simulink model "irep_force_control_simu"  (Simulink 8.5)
settings: Solver=ode3  StartTime=0.0  StopTime=inf  FixedStep=dt  RelTol=1e-3
InitFcn:
  | IREP_DEPENDENCY
  | init_omni
  | init_filters
  | init_invivo
  | init_telemanipulation
  | init_parker_xyz
  | init_magnetic_tracker
  | init_loadcell
  | init_scopes
  | init_homing
  | init_force_control
  | init_xpc_invivo_simu
undefined symbols (not defined in the file): ang_vel_scale, B_simu, beta, camera_home_voltage, counter_offset, dt, dt_trakstar, E_Y, encoder_counts, epsilon_robust_inverse, gear_ratio, HomingFineEps, HomingRoughEps, HomingRoughVelocity, I1_primary, I1_secondary, I2_primary, I2_secondary, irep_parameters_left, irep_parameters_right, joystick_filter_coeffs, K_d, K_i, K_naive_inv, K_p, k_right, L1l, L1r, L2l, L2r, L_zeus, left_arm_home_voltage, left_x0_parallelogram, LeftArmHomingDirectionVector, LeftArmHomingIntGain, lin_vel_scale, LOADCELL_BIAS, LOADCELL_GAIN, max_conf_space_speed, N_joystick, N_pots, N_trakstar, OmegaMax, OmegaMin, orientation_epsilon, position_epsilon, pots_filter_coeffs, q_eps_backlash, quadrature_mode, r, right_arm_home_voltage, RightArmHomingDirectionVector, RightArmHomingIntGain, screw_pitch, statics_param, tau_compression_bias, tau_compression_gains, tau_neutral_deadband, tau_tension_bias, tau_tension_gains ... (+14)
libraries: slrtlib x38, xpcrtudplib x13, xpcobsoletelib x13, simulink x6, dspswit3 x2, dspsigops x1
(part 2 of 6)

== system irep_force_control_simu/Joint Level PID Control in mm/PID Compensator ==
  e : Inport
  Enable : EnablePort  StatesWhenEnabling=reset
  Add : Sum  Inputs=+++
  Discrete Derivative : simulink/Discrete/Discrete Derivative  gainval=1.0  ICPrevScaledInput=0.0  InputProcessing=Inherited  OutMin=[]  OutMax=[]  OutDataType=sfix(16)  OutScaling=2^-10  DoSatur=off
  Discrete-Time Integrator : DiscreteIntegrator  SampleTime=dt
  Integral Sat : Saturate  UpperLimit=5  LowerLimit=-5
  Kd : Gain  Gain=K_d  SampleTime=dt
  Ki : Gain  Gain=K_i  SampleTime=dt
  Kp : Gain  Gain=K_p  SampleTime=dt
  Saturation : Saturate  UpperLimit=10  LowerLimit=-10
  u : Outport  InitialOutput=zeros(23,1)
  wires:
  Discrete Derivative/1 -> Add/3
  Kd/1 -> Discrete Derivative/1
  Integral Sat/1 -> Add/2
  Discrete-Time Integrator/1 -> Integral Sat/1
  Saturation/1 -> u/1
  Add/1 -> Saturation/1
  Ki/1 -> Discrete-Time Integrator/1
  Kp/1 -> Add/1
  e/1 -> Ki/1, Kp/1, Kd/1

== system irep_force_control_simu/Scopes/Friction Estimation Data UDP ==
  note: ConfigSpace:
      | b0 [1x1]
      | b1 [2x1]
      | psi [4x1]
      | gamma [1x1]
  note: [9x1]
  note: [4x1]
  note: [6x1]
  note: [6x1]
  note: [6x1]
  note: [6x1]
  sensors : Inport
  ConfigComd : Inport  Port=2
  Clock : Inport  Port=3
  Enable : EnablePort
  Bus Selector1 : BusSelector  OutputSignals=Magnetic Sensors.s1,Magnetic Sensors.s2,Magnetic Sensors.s3,Magnetic Sensors.s4
  Bus Selector2 : BusSelector  OutputSignals=force_sensing.loadcell
  Bus Selector4 : BusSelector  OutputSignals=A/D signals.right arm pots
  Demux : Demux  Outputs=[1 6 1]
  Demux1 : Demux  Outputs=54
  Demux2 : Demux  Outputs=[9 1]
  Mux : Mux  Inputs=10
  Pack : xpcobsoletelib/Utilities/Pack   datatypes={'double' 'double' 'double' 'double' 'double' 'double' 'double' 'double' 'double' 'double' 'double' 'double' 'double' 'double' 'double' 'double' 'double' 'double' 'double' 'double' 'double' 'double' 'double' 'double' 'double' 'double' 'double' 'double' 'double' 'double' 'double' 'double' 'double' 'double' 'double' 'double' 'double' 'double' 'double' 'double' 'double' 'double' 'double' 'double' 'double' 'double' 'double' 'double' 'double' 'double' 'double' 'double' 'double' 'double'}  byteAlign=1
  Rate Transition : RateTransition  OutPortSampleTime=0.012
  Right arm joint def : Subsystem
  STOP : Constant  Value=0
  Send port: 10001 : xpcrtudplib/Legacy UDP/Send   ipAddress=192.168.1.31  ipPort=10001  localPort=-1  vblLen=off  sampletime=0.01
  Terminator : Terminator
  Terminator1 : Terminator
  Terminator2 : Terminator
  wires:
  Pack/1 -> Send port: 10001/1
  sensors/1 -> Right arm joint def/1(sensors), Bus Selector4/1, Bus Selector2/1, Bus Selector1/1
  Bus Selector2/1 -> Mux/3  "<loadcell>"
  Bus Selector1/1 -> Mux/4  "<s1>"
  Bus Selector1/2 -> Mux/5  "<s2>"
  Bus Selector1/3 -> Mux/6  "<s3>"
  Bus Selector1/4 -> Mux/7  "<s4>"
  Right arm joint def/1(right q_cur) -> Mux/1  "q_cur [9x1]"
  ConfigComd/1 -> Demux/1
  Demux/1 -> Terminator/1
  Demux/2 -> Mux/8  "b,psi [6x1]"
  Clock/1 -> Mux/9  "clock [1x1]"
  Mux/1 -> Rate Transition/1
  Demux1/1 -> Pack/1
  Demux1/2 -> Pack/2
  Demux1/3 -> Pack/3
  Demux1/4 -> Pack/4
  Demux1/5 -> Pack/5
  Demux1/6 -> Pack/6
  Demux1/7 -> Pack/7
  Demux1/8 -> Pack/8
  Demux1/9 -> Pack/9
  Demux1/10 -> Pack/10
  Demux1/11 -> Pack/11
  Demux1/12 -> Pack/12
  Demux1/13 -> Pack/13
  Demux1/14 -> Pack/14
  Demux1/15 -> Pack/15
  Demux1/16 -> Pack/16
  Demux1/17 -> Pack/17
  Demux1/18 -> Pack/18
  Demux1/19 -> Pack/19
  Demux1/20 -> Pack/20
  Demux1/21 -> Pack/21
  Demux1/22 -> Pack/22
  Demux1/23 -> Pack/23
  Demux1/24 -> Pack/24
  Demux1/25 -> Pack/25
  Demux1/26 -> Pack/26
  Demux1/27 -> Pack/27
  Demux1/28 -> Pack/28
  Demux1/29 -> Pack/29
  Demux1/30 -> Pack/30
  Demux1/31 -> Pack/31
  Demux1/32 -> Pack/32
  Demux1/33 -> Pack/33
  Demux1/34 -> Pack/34
  Demux1/35 -> Pack/35
  Demux1/36 -> Pack/36
  Demux1/37 -> Pack/37
  Demux1/38 -> Pack/38
  Demux1/39 -> Pack/39
  Demux1/40 -> Pack/40
  Demux1/41 -> Pack/41
  Demux1/42 -> Pack/42
  Demux1/43 -> Pack/43
  Demux1/44 -> Pack/44
  Demux1/45 -> Pack/45
  Demux1/46 -> Pack/46
  Demux1/47 -> Pack/47
  Demux1/48 -> Pack/48
  Demux1/49 -> Pack/49
  Demux1/50 -> Pack/50
  Demux1/51 -> Pack/51
  Demux1/52 -> Pack/52
  Demux1/53 -> Pack/53
  Demux1/54 -> Pack/54
  Rate Transition/1 -> Demux1/1
  STOP/1 -> Mux/10
  Demux/3 -> Terminator1/1
  Bus Selector4/1 -> Demux2/1  "<right arm pots>"
  Demux2/1 -> Mux/2
  Demux2/2 -> Terminator2/1

== system irep_force_control_simu/Scopes/Left arm joint def ==
  In1 : Inport
  Bus Selector5 : BusSelector  OutputSignals=q.Left arm - overall translational movement,q.Left arm - parallelogram insert joint,q.Left arm - parallelogram deployment joint,q.Left arm - proximal segment - bending in X,q.Left arm - proximal segment - bending in Y,q.Left arm - distal segment - bending in x,q.Left arm - distal segment - bending in y,q.Left arm - wrist,q.Left arm - gripper joint
  Mux5 : Mux  Inputs=9
  Out1 : Outport
  wires:
  Bus Selector5/1 -> Mux5/1  "<Left arm - overall translational movement>"
  Bus Selector5/2 -> Mux5/2  "<Left arm - parallelogram insert joint>"
  Bus Selector5/3 -> Mux5/3  "<Left arm - parallelogram deployment joint>"
  Bus Selector5/4 -> Mux5/4  "<Left arm - proximal segment - bending in X>"
  Bus Selector5/5 -> Mux5/5  "<Left arm - proximal segment - bending in Y>"
  Bus Selector5/6 -> Mux5/6  "<Left arm - distal segment - bending in x>"
  Bus Selector5/7 -> Mux5/7  "<Left arm - distal segment - bending in y>"
  Bus Selector5/8 -> Mux5/8  "<Left arm - wrist>"
  Bus Selector5/9 -> Mux5/9  "<Left arm - gripper joint>"
  In1/1 -> Bus Selector5/1
  Mux5/1 -> Out1/1

== system irep_force_control_simu/Scopes/Magnetic Sensor Scopes ==
  In1 : Inport
  Bus Selector4 : BusSelector  OutputSignals=Magnetic Sensors.s1
  Bus Selector5 : BusSelector  OutputSignals=Magnetic Sensors.s2
  Bus Selector6 : BusSelector  OutputSignals=Magnetic Sensors.s3
  Bus Selector7 : BusSelector  OutputSignals=Magnetic Sensors.s4
  Scope M sensor 1 : slrtlib/Displays and Logging/Scope   scopeno=22  scopetype=Host  autostart=on  viewmode=Numerical  formatstr=scope_format_Msensor_1  grid=on  ylimits=[0,0]  nosamples=50  noprepostsamples=0  interleave=1  triggermode=FreeRun  triggersignal=1  trigsignalfromport=off  triggerlevel=0.0  triggerslope=Either  triggerscope=1  triggersample=0  filename=data.dat  mode=Lazy  writesize=512  autorestart=off  dynamicfilemode=off  maxwritefilesize=512*1024^2
  Scope M sensor 2 : slrtlib/Displays and Logging/Scope   scopeno=23  scopetype=Host  autostart=off  viewmode=Numerical  formatstr=scope_format_Msensor_2  grid=on  ylimits=[0,0]  nosamples=50  noprepostsamples=0  interleave=1  triggermode=FreeRun  triggersignal=1  trigsignalfromport=off  triggerlevel=0.0  triggerslope=Either  triggerscope=1  triggersample=0  filename=data.dat  mode=Lazy  writesize=512  autorestart=off  dynamicfilemode=off  maxwritefilesize=512*1024^2
  "Scope M sensor 3 " : slrtlib/Displays and Logging/Scope   scopeno=30  scopetype=Host  autostart=on  viewmode=Numerical  formatstr=scope_format_Msensor_3  grid=on  ylimits=[0,0]  nosamples=50  noprepostsamples=0  interleave=1  triggermode=FreeRun  triggersignal=1  trigsignalfromport=off  triggerlevel=0.0  triggerslope=Either  triggerscope=1  triggersample=0  filename=data.dat  mode=Lazy  writesize=512  autorestart=off  dynamicfilemode=off  maxwritefilesize=512*1024^2
  Scope M sensor 4 : slrtlib/Displays and Logging/Scope   scopeno=31  scopetype=Host  autostart=on  viewmode=Numerical  formatstr=scope_format_Msensor_4  grid=on  ylimits=[0,0]  nosamples=50  noprepostsamples=0  interleave=1  triggermode=FreeRun  triggersignal=1  trigsignalfromport=off  triggerlevel=0.0  triggerslope=Either  triggerscope=1  triggersample=0  filename=data.dat  mode=Lazy  writesize=512  autorestart=off  dynamicfilemode=off  maxwritefilesize=512*1024^2
  wires:
  Bus Selector4/1 -> Scope M sensor 1/1  "<s1>"
  Bus Selector5/1 -> Scope M sensor 2/1  "<s2>"
  Bus Selector6/1 -> "Scope M sensor 3 "/1  "<s3>"
  Bus Selector7/1 -> Scope M sensor 4/1  "<s4>"
  In1/1 -> Bus Selector4/1, Bus Selector6/1, Bus Selector5/1, Bus Selector7/1

== system irep_force_control_simu/Scopes/Other_scope ==
  In1 : Inport
  Bus Selector2 : BusSelector  OutputSignals=A/D signals.right arm pots,A/D signals.left arm pots,q.Parker insertion stage,q.Parker rotary stage,q.Camera shell open,q.Camera Pan,q.Camera Tilt,foot switches,Pots_Connect
  Camera : slrtlib/Displays and Logging/Scope   scopeno=6  scopetype=Host  autostart=on  viewmode=Numerical  formatstr='Camera: %3.3f'  grid=on  ylimits=[0,0]  nosamples=10  noprepostsamples=0  interleave=1  triggermode=FreeRun  triggersignal=1  trigsignalfromport=off  triggerlevel=0.0  triggerslope=Either  triggerscope=1  triggersample=0  filename=weights1.dat  mode=Lazy  writesize=512  autorestart=off  dynamicfilemode=off  maxwritefilesize=512*1024^2
  Digital Input : slrtlib/Displays and Logging/Scope   scopeno=2  scopetype=Host  autostart=on  viewmode=Numerical  formatstr=scope_format_digital_input  grid=on  ylimits=[0,0]  nosamples=10  noprepostsamples=0  interleave=1  triggermode=FreeRun  triggersignal=1  trigsignalfromport=off  triggerlevel=0.0  triggerslope=Either  triggerscope=1  triggersample=0  filename=weights1.dat  mode=Lazy  writesize=512  autorestart=off  dynamicfilemode=off  maxwritefilesize=512*1024^2
  Left Arm Pots : slrtlib/Displays and Logging/Scope   scopeno=7  scopetype=Target  autostart=on  viewmode=Numerical  formatstr=scope_format_left_pot  grid=on  ylimits=[0,0]  nosamples=10  noprepostsamples=0  interleave=1  triggermode=FreeRun  triggersignal=1  trigsignalfromport=off  triggerlevel=0.0  triggerslope=Either  triggerscope=1  triggersample=0  filename=weights1.dat  mode=Lazy  writesize=512  autorestart=off  dynamicfilemode=off  maxwritefilesize=512*1024^2
  Mux2 : Mux  Inputs=2
  Mux3 : Mux  Inputs=3
  Mux4 : Mux  Inputs=2
  Parker Feedback : slrtlib/Displays and Logging/Scope   scopeno=4  scopetype=Host  autostart=on  viewmode=Numerical  formatstr=scope_format_parker_cur  grid=on  ylimits=[0,0]  nosamples=10  noprepostsamples=0  interleave=1  triggermode=FreeRun  triggersignal=1  trigsignalfromport=off  triggerlevel=0.0  triggerslope=Either  triggerscope=1  triggersample=0  filename=weights1.dat  mode=Lazy  writesize=512  autorestart=off  dynamicfilemode=off  maxwritefilesize=512*1024^2
  Right Arm Pots : slrtlib/Displays and Logging/Scope   scopeno=8  scopetype=Host  autostart=on  viewmode=Numerical  formatstr=scope_format_right_pot  grid=on  ylimits=[0,0]  nosamples=10  noprepostsamples=0  interleave=1  triggermode=FreeRun  triggersignal=1  trigsignalfromport=off  triggerlevel=0.0  triggerslope=Either  triggerscope=1  triggersample=0  filename=weights1.dat  mode=Lazy  writesize=512  autorestart=off  dynamicfilemode=off  maxwritefilesize=512*1024^2
  wires:
  Bus Selector2/1 -> Right Arm Pots/1  "<right arm pots>"
  Bus Selector2/2 -> Left Arm Pots/1  "<left arm pots>"
  Bus Selector2/3 -> Mux2/1  "<Parker insertion stage>"
  Bus Selector2/4 -> Mux2/2  "<Parker rotary stage>"
  Mux2/1 -> Parker Feedback/1
  Mux3/1 -> Camera/1
  Bus Selector2/5 -> Mux3/1  "<Camera shell open>"
  Bus Selector2/6 -> Mux3/2  "<Camera Pan>"
  Bus Selector2/7 -> Mux3/3  "<Camera Tilt>"
  Bus Selector2/8 -> Mux4/1  "<foot switches>"
  Bus Selector2/9 -> Mux4/2  "<Pots_Connect>"
  Mux4/1 -> Digital Input/1
  In1/1 -> Bus Selector2/1

== system irep_force_control_simu/Scopes/Right arm joint def ==
  In1 : Inport
  Bus Selector4 : BusSelector  OutputSignals=q.Right arm - overall translational movement,q.Right arm - parallelogram insert joint,q.Right arm - parallelogram deployment joint,q.Right arm - Proximal segment - bending in X,q.Righ arm - Proximal segment - bending in Y,q.Right arm - distal segment - bending in X,q.Right arm - distal segment - bending in Y,q.Right arm - wrist,q.Right arm - Gripper Joint
  Mux1 : Mux  Inputs=9
  Out1 : Outport
  wires:
  Bus Selector4/1 -> Mux1/1  "<Right arm - overall translational movement>"
  Bus Selector4/2 -> Mux1/2  "<Right arm - parallelogram insert joint>"
  Bus Selector4/3 -> Mux1/3  "<Right arm - parallelogram deployment joint>"
  Bus Selector4/4 -> Mux1/4  "<Right arm - Proximal segment - bending in X>"
  Bus Selector4/5 -> Mux1/5  "<Righ arm - Proximal segment - bending in Y>"
  Bus Selector4/6 -> Mux1/6  "<Right arm - distal segment - bending in X>"
  Bus Selector4/7 -> Mux1/7  "<Right arm - distal segment - bending in Y>"
  Bus Selector4/8 -> Mux1/8  "<Right arm - wrist>"
  Bus Selector4/9 -> Mux1/9  "<Right arm - Gripper Joint>"
  In1/1 -> Bus Selector4/1
  Mux1/1 -> Out1/1

== system irep_force_control_simu/Scopes/left ==
  In1 : Inport
  Bus Selector : BusSelector  OutputSignals=Left arm - Proximal Segment Y,Left arm - Gripper Joint,Left arm - Proximal Segment X,Left arm - Distal Segment X,Left arm - Wrist Joint,Left arm - Distal Segment Y,Left arm - Parallelogram Deploy,Left arm - Parallelogram Insert,Left arm - Overall Translational Movement
  Gain{1..4} (4 alike) : Gain  Gain=-1
  Mux : Mux  Inputs=9
  Out1 : Outport
  wires:
  Bus Selector/1 -> Gain1/1  "<Left arm - Proximal Segment Y>"
  Bus Selector/2 -> Mux/2  "<Left arm - Gripper Joint>"
  Bus Selector/4 -> Mux/4  "<Left arm - Distal Segment X>"
  Bus Selector/5 -> Mux/5  "<Left arm - Wrist Joint>"
  Bus Selector/6 -> Gain2/1  "<Left arm - Distal Segment Y>"
  Bus Selector/7 -> Gain3/1  "<Left arm - Parallelogram Deploy>"
  Bus Selector/8 -> Gain4/1  "<Left arm - Parallelogram Insert>"
  In1/1 -> Bus Selector/1
  Mux/1 -> Out1/1
  Bus Selector/3 -> Mux/3  "<Left arm - Proximal Segment X>"
  Gain1/1 -> Mux/1
  Gain2/1 -> Mux/6
  Gain3/1 -> Mux/7
  Gain4/1 -> Mux/8
  Bus Selector/9 -> Mux/9  "<Left arm - Overall Translational Movement>"

== system irep_force_control_simu/Scopes/parker ==
  In1 : Inport
  Bus Selector : BusSelector  OutputSignals=Parker insertion stage,Parker rotary stage
  Gain1 : Gain  Gain=-1
  Gain2 : Gain  Gain=-1
  Mux : Mux  Inputs=2
  Out1 : Outport
  wires:
  Bus Selector/1 -> Gain1/1  "<Parker insertion stage>"
  Bus Selector/2 -> Gain2/1  "<Parker rotary stage>"
  In1/1 -> Bus Selector/1
  Mux/1 -> Out1/1
  Gain1/1 -> Mux/1
  Gain2/1 -> Mux/2

== system irep_force_control_simu/Scopes/right ==
  In1 : Inport
  Bus Selector : BusSelector  OutputSignals=Right arm - Proximal Segment Y,Right arm - Gripper Joint,Right arm - Proximal Segment X,Right arm - Distal Segment X,Right arm - Wrist Joint,Right arm - Distal Segment Y,Right arm - Parallelogram Deploy,Right arm - Parallelogram Insert,Righ arm - Overall Translational Movement
  Mux : Mux  Inputs=9
  Out1 : Outport
  wires:
  In1/1 -> Bus Selector/1
  Mux/1 -> Out1/1
  Bus Selector/3 -> Mux/3  "<Right arm - Proximal Segment X>"
  Bus Selector/4 -> Mux/4  "<Right arm - Distal Segment X>"
  Bus Selector/5 -> Mux/5  "<Right arm - Wrist Joint>"
  Bus Selector/6 -> Mux/6  "<Right arm - Distal Segment Y>"
  Bus Selector/8 -> Mux/8  "<Right arm - Parallelogram Insert>"
  Bus Selector/2 -> Mux/2  "<Right arm - Gripper Joint>"
  Bus Selector/1 -> Mux/1  "<Right arm - Proximal Segment Y>"
  Bus Selector/7 -> Mux/7  "<Right arm - Parallelogram Deploy>"
  Bus Selector/9 -> Mux/9  "<Righ arm - Overall Translational Movement>"

== system irep_force_control_simu/Scopes/select wrench ==
  In : Inport
  Bus Selector4 : BusSelector  OutputSignals=Ws_right,We_right_seg1
  Demux : Demux  Outputs=[3,3]
  Demux1 : Demux  Outputs=[3,3]
  Mux : Mux  Inputs=2
  Terminator : Terminator
  Terminator1 : Terminator
  Out : Outport
  wires:
  Bus Selector4/1 -> Demux/1  "<Ws_right>"
  Bus Selector4/2 -> Demux1/1  "<We_right_seg1>"
  Demux/2 -> Terminator/1  "Torque"
  Demux1/2 -> Terminator1/1  "Torque"
  Demux/1 -> Mux/1  "Force"
  Demux1/1 -> Mux/2  "Force"
  Mux/1 -> Out/1
  In/1 -> Bus Selector4/1

== system irep_force_control_simu/Trajectory Planner/Camera ==
  vision : Inport
  sensors : Inport  Port=2
  Enable : EnablePort
  Enable Homing : Constant  Value=0  SampleTime=dt
  Enable Joint Space : Constant  Value=0  SampleTime=dt
  Enable Joystick : Constant  Value=0  SampleTime=dt
  Enable Tool Tracking : Constant  Value=0  SampleTime=dt
  Homing Procedure : Subsystem  TreatAsAtomicUnit=on
  Joint Space : Subsystem  TreatAsAtomicUnit=on
  Joystick Control for Cam : Subsystem  TreatAsAtomicUnit=on
  Merge : Merge  Inputs=4  InitialOutput=zeros(3,1)
  Saturation : Saturate  UpperLimit=[5 1.6 1.5]  LowerLimit=[-5 -1.6 -1.5]
  Tool Tracking : Subsystem  TreatAsAtomicUnit=on
  q des camera : Outport  InitialOutput=zeros(3,1)
  wires:
  Enable Tool Tracking/1 -> Tool Tracking/Enable
  Merge/1 -> Saturation/1
  vision/1 -> Tool Tracking/1(tool XY)
  Enable Joint Space/1 -> Joint Space/Enable
  sensors/1 -> Joystick Control for Cam/1(sensors), Homing Procedure/1(sensors)
  Enable Joystick/1 -> Joystick Control for Cam/Enable
  Homing Procedure/1(q des) -> Merge/1
  Joint Space/1(Out1) -> Merge/2
  Tool Tracking/1(q des) -> Merge/3
  Joystick Control for Cam/1(q des) -> Merge/4
  Enable Homing/1 -> Homing Procedure/Enable
  Saturation/1 -> q des camera/1

== system irep_force_control_simu/Trajectory Planner/Delay_test ==
  Delay_test : xpcrtudplib/Legacy UDP/Send   ipAddress=192.168.1.64  ipPort=10031  localPort=-1  vblLen=off  sampletime=0.01
  Digital Clock : DigitalClock  SampleTime=dt
  Pack1 : xpcobsoletelib/Utilities/Pack   datatypes={'double'}  byteAlign=1
  Receive : xpcrtudplib/Legacy UDP/Receive   ipAddress=0.0.0.0  ipPort=10030  width=8  vblLen=on  sampletime=0.01
  "Scope (xPC) " : slrtlib/Displays and Logging/Scope   scopeno=25  scopetype=Host  autostart=on  viewmode=Numerical  formatstr='Delay:%15.6f'  grid=on  ylimits=[0,0]  nosamples=250  noprepostsamples=0  interleave=1  triggermode=FreeRun  triggersignal=1  trigsignalfromport=off  triggerlevel=0.0  triggerslope=Either  triggerscope=1  triggersample=0  filename=data.dat  mode=Lazy  writesize=512  autorestart=off  dynamicfilemode=off  maxwritefilesize=512*1024^2
  Sum : Sum  Inputs=|+-
  Terminator : Terminator
  Unpack : xpcobsoletelib/Utilities/Unpack   dimensions={1}  datatypes={'double'}  byteAlign=1
  wires:
  Digital Clock/1 -> Pack1/1, Sum/1
  Pack1/1 -> Delay_test/1
  Receive/2 -> Terminator/1
  Receive/1 -> Unpack/1
  Unpack/1 -> Sum/2
  Sum/1 -> "Scope (xPC) "/1

== system irep_force_control_simu/Trajectory Planner/Left Arm ==
  note: IREP Left Arm Trajectory Planner - v 0.6 - © COPYRIGHT 2011 Andrea Bajo, Nabil Simaan
  Master : Inport
  sensors : Inport  Port=2
  Enable : EnablePort
  Enable High Level : Constant  Value=0  SampleTime=dt
  Enable Low Level : Constant  Value=0  SampleTime=dt
  High Level : Subsystem  TreatAsAtomicUnit=on
  Low Level : Subsystem  TreatAsAtomicUnit=on
  Merge1 : Merge  InitialOutput=zeros(9,1)
  q left arm : Outport  InitialOutput=zeros(9,1)
  conf space : Outport  Port=2
  b0 dot left : Outport  Port=3
  TASK_EN : Outport  Port=4
  current_pose : Outport  Port=5
  wires:
  Enable Low Level/1 -> Low Level/Enable
  Low Level/1(q des) -> Merge1/1
  Enable High Level/1 -> High Level/Enable
  High Level/1(q des) -> Merge1/2
  sensors/1 -> Low Level/1(sensors), High Level/2(sensors)
  Master/1 -> High Level/1(Master)
  Merge1/1 -> q left arm/1
  High Level/2(conf space) -> conf space/1
  High Level/3(b0_dot_left) -> b0 dot left/1
  High Level/4(TASK_EN) -> TASK_EN/1
  High Level/5(current_pose) -> current_pose/1

== system irep_force_control_simu/Trajectory Planner/RZ ==
  trajectory : Inport
  sensors : Inport  Port=2
  Enable : EnablePort
  Add : Sum
  Arm selector : MATLAB Function  TreatAsAtomicUnit=on
  Bus Selector1 : BusSelector  OutputSignals=right arm.b0 dot right,left arm.b0 dot left
  Discrete-Time Integrator : DiscreteIntegrator  InitialCondition=[0;0]  SampleTime=dt  LimitOutput=on  UpperSaturationLimit=[200;pi/2]  LowerSaturationLimit=[-100;0]
  Enable Joint Space : Constant  Value=0  SampleTime=dt
  Joystick Control for RZ : Subsystem  TreatAsAtomicUnit=on
  Subsystem : Subsystem
  Parker : Outport  InitialOutput=zeros(2,1)
  wires:
  sensors/1 -> Joystick Control for RZ/1(sensors)
  Joystick Control for RZ/1(q des) -> Subsystem/1(In1)
  Enable Joint Space/1 -> Joystick Control for RZ/Enable
  Add/1 -> Discrete-Time Integrator/1
  Subsystem/1(Out1) -> Add/2
  Arm selector/1(b0dot) -> Add/1
  Discrete-Time Integrator/1 -> Parker/1
  trajectory/1 -> Bus Selector1/1
  Bus Selector1/1 -> Arm selector/1(right_b0_dot)  "<b0 dot right>"
  Bus Selector1/2 -> Arm selector/2(left_b0_dot)  "<b0 dot left>"

== system irep_force_control_simu/Trajectory Planner/Right Arm ==
  note: IREP Right Arm Trajectory Planner - v 1.0 - © COPYRIGHT 2011 Andrea Bajo, Nabil Simaan
  Master : Inport
  sensors : Inport  Port=2
  Enable : EnablePort
  Enable High Level : Constant  Value=0  SampleTime=dt
  Enable Low Level : Constant  Value=0  SampleTime=dt
  High Level : Subsystem  TreatAsAtomicUnit=on
  Low Level : Subsystem  TreatAsAtomicUnit=on
  Merge1 : Merge  InitialOutput=zeros(9,1)
  conf space : Outport  PortDimensions=8
  q right arm : Outport  Port=2  InitialOutput=zeros(9,1)
  b0 dot right : Outport  Port=3
  TASK_EN : Outport  Port=4
  current_pose : Outport  Port=5
  wires:
  Enable Low Level/1 -> Low Level/Enable
  Low Level/1(q des) -> Merge1/1
  Enable High Level/1 -> High Level/Enable
  High Level/1(q des) -> Merge1/2
  sensors/1 -> Low Level/1(sensors), High Level/2(sensors)
  Master/1 -> High Level/1(Master)
  High Level/2(conf space) -> conf space/1
  High Level/3(b0 dot) -> b0 dot right/1
  High Level/4(TASK_EN) -> TASK_EN/1
  Merge1/1 -> q right arm/1
  High Level/5(current_pose) -> current_pose/1

== system irep_force_control_simu/Trajectory Planner/Signals packing ==
  irep : Inport
  parker : Inport  Port=2
  Bus Creator : BusCreator
  Bus Selector : BusSelector  OutputSignals=right arm.q des right,left arm.q des left,camera q
  system : Outport
  wires:
  Bus Selector/1 -> Bus Creator/1  "<q des right>"
  Bus Selector/2 -> Bus Creator/2  "<q des left>"
  Bus Selector/3 -> Bus Creator/3  "<camera q>"
  irep/1 -> Bus Selector/1
  Bus Creator/1 -> system/1
  parker/1 -> Bus Creator/4

== system irep_force_control_simu/Trajectory Planner/UDP_SendTo_MTM ==
  Traj : Inport
  Right_MTM : Inport  Port=2
  Left_MTM : Inport  Port=3
  Right_Wrench : Inport  Port=4
  Left_UDP : Subsystem
  Right_UDP : Subsystem
  wires:
  Traj/1 -> Right_UDP/1(traj), Left_UDP/1(traj)
  Right_MTM/1 -> Right_UDP/2(MTM)
  Left_MTM/1 -> Left_UDP/2(MTM)
  Right_Wrench/1 -> Right_UDP/3(Wrench)

== system irep_force_control_simu/Wrench Estimation/combine psi ==
  note: Combining measured psi and commanded psi
      | measured psi has a good estimate of theta
      | but very poor estimate of delta
  psi_m : Inport
  psi_d : Inport  Port=2
  Bus Selector : BusSelector  OutputSignals=right arm.right arm conf space.psi curr
  Demux : Demux  Outputs=[4,1]
  Gain : Gain  Gain=[1,0,1,0]
  Gain1 : Gain  Gain=[0,1,0,1]
  Sum : Sum  Inputs=|++
  Terminator : Terminator
  psi : Outport
  wires:
  psi_m/1 -> Gain/1
  Sum/1 -> psi/1
  psi_d/1 -> Bus Selector/1
  Bus Selector/1 -> Demux/1  "<psi curr>"
  Demux/2 -> Terminator/1
  Demux/1 -> Gain1/1
  Gain/1 -> Sum/1
  Gain1/1 -> Sum/2

== system irep_force_control_simu/Wrench Estimation/q_cur to q_bb ==
  q_cur : Inport
  Bus Selector1 : BusSelector  OutputSignals=q.Right arm - Proximal segment - bending in X,q.Righ arm - Proximal segment - bending in Y,q.Right arm - distal segment - bending in X,q.Right arm - distal segment - bending in Y
  Gain{,1..3} (4 alike) : Gain  Gain=-1
  Mux1 : Mux  Inputs=8
  q_bb : Outport
  wires:
  q_cur/1 -> Bus Selector1/1
  Mux1/1 -> q_bb/1
  Bus Selector1/1 -> Mux1/1, Gain/1  "<Right arm - Proximal segment - bending in X>"
  Bus Selector1/2 -> Mux1/2, Gain1/1  "<Righ arm - Proximal segment - bending in Y>"
  Bus Selector1/3 -> Mux1/5, Gain2/1  "<Right arm - distal segment - bending in X>"
  Bus Selector1/4 -> Mux1/6, Gain3/1  "<Right arm - distal segment - bending in Y>"
  Gain/1 -> Mux1/3
  Gain1/1 -> Mux1/4
  Gain2/1 -> Mux1/7
  Gain3/1 -> Mux1/8

== system irep_force_control_simu/Wrench Estimation/sel param ==
  note: irep_parameters_right = [Y_OFFSET;L1r;L2r;p_gripper];
  In : Inport
  Demux : Demux  Outputs=[1,1,1,3]
  Mux1 : Mux  Inputs=2
  Terminator : Terminator
  Terminator1 : Terminator
  L : Outport
  wires:
  In/1 -> Demux/1
  Mux1/1 -> L/1
  Demux/2 -> Mux1/1  "L1"
  Demux/3 -> Mux1/2  "L2"
  Demux/1 -> Terminator/1  "Y_OFFSET"
  Demux/4 -> Terminator1/1  "p_gripper"

== system irep_force_control_simu/Wrench Estimation/tau sensing compensation ==
  q_bb : Inport
  tau_sensed : Inport  Port=2
  friction compensation : MATLAB Function  TreatAsAtomicUnit=on
  tau_compression_bias : Constant  Value=tau_compression_bias
  tau_compression_gains : Constant  Value=tau_compression_gains
  tau_neutral_deadband : Constant  Value=tau_neutral_deadband
  tau_tension_bias : Constant  Value=tau_tension_bias
  tau_tension_gains : Constant  Value=tau_tension_gains
  tau_comp : Outport
  wires:
  tau_neutral_deadband/1 -> friction compensation/7(deadband)
  tau_compression_gains/1 -> friction compensation/4(gain_compression)
  tau_tension_gains/1 -> friction compensation/3(gain_tension)
  tau_sensed/1 -> friction compensation/2(tau_sensed)
  q_bb/1 -> friction compensation/1(q_bb)
  friction compensation/1(tau_comp) -> tau_comp/1
  tau_tension_bias/1 -> friction compensation/5(bias_tension)
  tau_compression_bias/1 -> friction compensation/6(bias_compression)

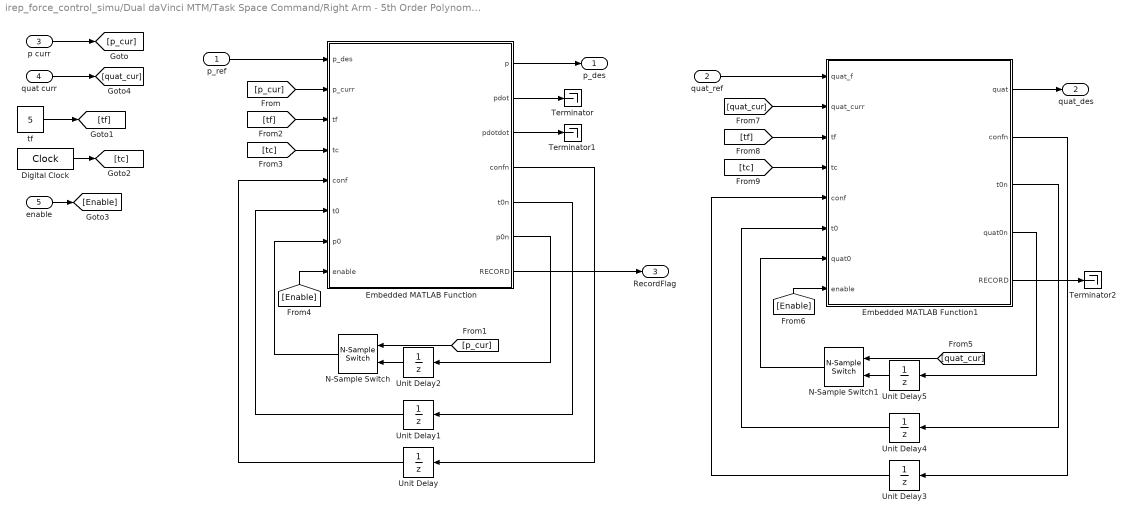
== system irep_force_control_simu/Dual daVinci MTM/Task Space Command/Right Arm - 5th Order Polynomial and Slerp ==
  p_ref : Inport
  quat_ref : Inport  Port=2
  p curr : Inport  Port=3
  quat curr : Inport  Port=4
  enable : Inport  Port=5
  Digital Clock : DigitalClock  SampleTime=dt
  Embedded MATLAB Function : MATLAB Function  TreatAsAtomicUnit=on
  Embedded MATLAB Function1 : MATLAB Function  TreatAsAtomicUnit=on
  N-Sample Switch : dspswit3/N-Sample Switch  N=1  reset=off  TriggerType=Rising edge  Ts=dt
  N-Sample Switch1 : dspswit3/N-Sample Switch  N=1  reset=off  TriggerType=Rising edge  Ts=dt
  Terminator : Terminator
  Terminator1 : Terminator
  Terminator2 : Terminator
  Unit Delay{,1..4} (5 alike) : UnitDelay  SampleTime=dt
  Unit Delay5 : UnitDelay  InitialCondition=[1;0;0;0]  SampleTime=dt
  tf : Constant  Value=5  SampleTime=dt
  p_des : Outport
  quat_des : Outport  Port=2
  RecordFlag : Outport  Port=3
  wires:
  Embedded MATLAB Function/4(confn) -> Unit Delay/1
  Unit Delay/1 -> Embedded MATLAB Function/5(conf)
  Embedded MATLAB Function/5(t0n) -> Unit Delay1/1
  Embedded MATLAB Function/6(p0n) -> Unit Delay2/1
  Unit Delay1/1 -> Embedded MATLAB Function/6(t0)
  p_ref/1 -> Embedded MATLAB Function/1(p_des)
  Embedded MATLAB Function/2(pdot) -> Terminator/1
  Embedded MATLAB Function/3(pdotdot) -> Terminator1/1
  N-Sample Switch/1 -> Embedded MATLAB Function/7(p0)
  Unit Delay2/1 -> N-Sample Switch/2
  p curr/1 -> [p_cur]
  [p_cur] -> Embedded MATLAB Function/2(p_curr)
  [p_cur] -> N-Sample Switch/1
  Embedded MATLAB Function/7(RECORD) -> RecordFlag/1
  Embedded MATLAB Function/1(p) -> p_des/1
  tf/1 -> [tf]
  Digital Clock/1 -> [tc]
  [tf] -> Embedded MATLAB Function/3(tf)
  [tc] -> Embedded MATLAB Function/4(tc)
  enable/1 -> [Enable]
  [Enable] -> Embedded MATLAB Function/8(enable)
  quat_ref/1 -> Embedded MATLAB Function1/1(quat_f)
  quat curr/1 -> [quat_cur]
  Embedded MATLAB Function1/3(t0n) -> Unit Delay4/1
  Embedded MATLAB Function1/4(quat0n) -> Unit Delay5/1
  Unit Delay4/1 -> Embedded MATLAB Function1/6(t0)
  N-Sample Switch1/1 -> Embedded MATLAB Function1/7(quat0)
  Unit Delay5/1 -> N-Sample Switch1/2
  [quat_cur] -> N-Sample Switch1/1
  Embedded MATLAB Function1/2(confn) -> Unit Delay3/1
  Unit Delay3/1 -> Embedded MATLAB Function1/5(conf)
  [Enable] -> Embedded MATLAB Function1/8(enable)
  [quat_cur] -> Embedded MATLAB Function1/2(quat_curr)
  [tf] -> Embedded MATLAB Function1/3(tf)
  [tc] -> Embedded MATLAB Function1/4(tc)
  Embedded MATLAB Function1/1(quat) -> quat_des/1
  Embedded MATLAB Function1/5(RECORD) -> Terminator2/1

== system irep_force_control_simu/Dual daVinci MTM/scopes/to file ==
  right : Inport
  left : Inport  Port=2
  Enable : EnablePort
  Joint Space Info File : slrtlib/Displays and Logging/Scope   scopeno=24  scopetype=File  autostart=on  viewmode=Numerical  formatstr="'tau: %8.3f,     %8.3f,     %8.3f,     %8.3f,     %8.3f,     %8.3f'"  grid=on  ylimits=[0,0]  nosamples=100000  noprepostsamples=0  interleave=1  triggermode=FreeRun  triggersignal=1  trigsignalfromport=off  triggerlevel=0.0  triggerslope=Either  triggerscope=1  triggersample=0  filename=MTMR.dat  mode=Lazy  writesize=512  autorestart=off  dynamicfilemode=off  maxwritefilesize=512*1024^2
  Terminator : Terminator
  wires:
  right/1 -> Joint Space Info File/1
  left/1 -> Terminator/1

== system irep_force_control_simu/In-Vivo System/CONTEC CARDS/Level 1 ==
  note: Contec
      | CNT32-8M (PCI)
      | Inc. Encoder
      | Slot: [1, 13]
  Constant{,1..7} (8 alike) : Constant  Value=0
  Mux : Mux  Inputs=8
  Out1 : Outport
  wires:
  Mux/1 -> Out1/1
  Constant/1 -> Mux/1
  Constant1/1 -> Mux/2
  Constant2/1 -> Mux/3
  Constant3/1 -> Mux/4
  Constant4/1 -> Mux/5
  Constant5/1 -> Mux/6
  Constant6/1 -> Mux/7
  Constant7/1 -> Mux/8

== system irep_force_control_simu/In-Vivo System/CONTEC CARDS/Level 2 ==
  note: Contec
      | CNT32-8M (PCI)
      | Inc. Encoder
      | Slot: [2, 8]
  Constant{,1..7} (8 alike) : Constant  Value=0
  Mux : Mux  Inputs=8
  Out1 : Outport
  wires:
  Mux/1 -> Out1/1
  Constant/1 -> Mux/1
  Constant1/1 -> Mux/2
  Constant2/1 -> Mux/3
  Constant3/1 -> Mux/4
  Constant4/1 -> Mux/5
  Constant5/1 -> Mux/6
  Constant6/1 -> Mux/7
  Constant7/1 -> Mux/8

== system irep_force_control_simu/In-Vivo System/CONTEC CARDS/Level 3 ==
  note: Contec
      | CNT32-8M (PCI)
      | Inc. Encoder
      | Slot: [2, 11]
      | channel [1,4,5,6,7]
  Constant{,1..4} (5 alike) : Constant  Value=0
  Mux : Mux  Inputs=5
  Out1 : Outport
  wires:
  Mux/1 -> Out1/1
  Constant/1 -> Mux/1
  Constant1/1 -> Mux/2
  Constant2/1 -> Mux/3
  Constant3/1 -> Mux/4
  Constant4/1 -> Mux/5

== system irep_force_control_simu/In-Vivo System/CONTEC CARDS/RZ ==
  note: Contec
      | CNT32-8M (PCI)
      | Inc. Encoder
      | Slot: [2, 14]
      | channel [1,2]
  Constant3 : Constant  Value=0
  Constant4 : Constant  Value=0
  Mux : Mux  Inputs=2
  Out1 : Outport
  wires:
  Constant4/1 -> Mux/2
  Constant3/1 -> Mux/1
  Mux/1 -> Out1/1

== system irep_force_control_simu/In-Vivo System/Count to mm/Bus Creator ==
  In1 : Inport
  Bus Creator : BusCreator  Inputs=23
  Demux : Demux  Outputs=23
  Out1 : Outport
  wires:
  Demux/1 -> Bus Creator/1  "Righ arm - Proximal segment - bending in Y"
  Demux/2 -> Bus Creator/2  "Right arm - Gripper Joint"
  Demux/3 -> Bus Creator/3  "Right arm - Proximal segment - bending in X"
  Demux/4 -> Bus Creator/4  "Right arm - distal segment - bending in X"
  Demux/5 -> Bus Creator/5  "Right arm - wrist"
  Demux/6 -> Bus Creator/6  "Right arm - distal segment - bending in Y"
  Demux/7 -> Bus Creator/7  "Right arm - parallelogram deployment joint"
  Demux/8 -> Bus Creator/8  "Right arm - parallelogram insert joint"
  Demux/9 -> Bus Creator/9  "Left arm - proximal segment - bending in Y"
  Demux/10 -> Bus Creator/10  "Left arm - gripper joint"
  Demux/11 -> Bus Creator/11  "Left arm - proximal segment - bending in X"
  Demux/12 -> Bus Creator/12  "Left arm - distal segment - bending in x"
  Demux/13 -> Bus Creator/13  "Left arm - wrist"
  Demux/14 -> Bus Creator/14  "Left arm - distal segment - bending in y"
  Demux/15 -> Bus Creator/15  "Left arm - parallelogram deployment joint"
  Demux/16 -> Bus Creator/16  "Left arm - parallelogram insert joint"
  Demux/17 -> Bus Creator/17  "Right arm - overall translational movement"
  Demux/18 -> Bus Creator/18  "Left arm - overall translational movement"
  Demux/19 -> Bus Creator/19  "Camera shell open"
  Demux/20 -> Bus Creator/20  "Camera Pan"
  Demux/21 -> Bus Creator/21  "Camera Tilt"
  Bus Creator/1 -> Out1/1
  In1/1 -> Demux/1
  Demux/22 -> Bus Creator/22  "Parker insertion stage"
  Demux/23 -> Bus Creator/23  "Parker rotary stage"

== system irep_force_control_simu/In-Vivo System/D/A/Bus Selector 1 ==
  In1 : Inport
  Bus Selector : BusSelector  OutputSignals=Right arm - Proximal Segment Y,Right arm - Gripper Joint,Right arm - Proximal Segment X,Right arm - Distal Segment X,Right arm - Wrist Joint,Right arm - Distal Segment Y,Right arm - Parallelogram Deploy,Right arm - Parallelogram Insert
  Gain{,1..3} (4 alike) : Gain  Gain=-1
  Mux : Mux  Inputs=8
  Out1 : Outport
  wires:
  Bus Selector/1 -> Mux/1  "<Right arm - Proximal Segment Y>"
  Bus Selector/2 -> Mux/2  "<Right arm - Gripper Joint>"
  Bus Selector/3 -> Gain/1  "<Right arm - Proximal Segment X>"
  Bus Selector/4 -> Gain1/1  "<Right arm - Distal Segment X>"
  Bus Selector/5 -> Mux/5  "<Right arm - Wrist Joint>"
  Bus Selector/6 -> Mux/6  "<Right arm - Distal Segment Y>"
  Bus Selector/7 -> Gain2/1  "<Right arm - Parallelogram Deploy>"
  Bus Selector/8 -> Gain3/1  "<Right arm - Parallelogram Insert>"
  In1/1 -> Bus Selector/1
  Mux/1 -> Out1/1
  Gain/1 -> Mux/3
  Gain1/1 -> Mux/4
  Gain2/1 -> Mux/7
  Gain3/1 -> Mux/8

== system irep_force_control_simu/In-Vivo System/D/A/Bus Selector 2 ==
  In1 : Inport
  Bus Selector : BusSelector  OutputSignals=Left arm - Proximal Segment Y,Left arm - Gripper Joint,Left arm - Proximal Segment X,Left arm - Distal Segment X,Left arm - Wrist Joint,Left arm - Distal Segment Y,Left arm - Parallelogram Deploy,Left arm - Parallelogram Insert
  Gain{1..4} (4 alike) : Gain  Gain=-1
  Mux : Mux  Inputs=8
  Out1 : Outport
  wires:
  Bus Selector/1 -> Gain1/1  "<Left arm - Proximal Segment Y>"
  Bus Selector/2 -> Mux/2  "<Left arm - Gripper Joint>"
  Bus Selector/4 -> Mux/4  "<Left arm - Distal Segment X>"
  Bus Selector/5 -> Mux/5  "<Left arm - Wrist Joint>"
  Bus Selector/6 -> Gain2/1  "<Left arm - Distal Segment Y>"
  Bus Selector/7 -> Gain3/1  "<Left arm - Parallelogram Deploy>"
  Bus Selector/8 -> Gain4/1  "<Left arm - Parallelogram Insert>"
  In1/1 -> Bus Selector/1
  Mux/1 -> Out1/1
  Bus Selector/3 -> Mux/3  "<Left arm - Proximal Segment X>"
  Gain1/1 -> Mux/1
  Gain2/1 -> Mux/6
  Gain3/1 -> Mux/7
  Gain4/1 -> Mux/8

== system irep_force_control_simu/In-Vivo System/D/A/Bus Selector 3 ==
  In1 : Inport
  Bus Selector : BusSelector  OutputSignals=Righ arm - Overall Translational Movement,Left arm - Overall Translational Movement,Camera shell open,Camera Pan,Camera Tilt
  Mux : Mux  Inputs=5
  Out1 : Outport
  wires:
  Mux/1 -> Out1/1
  In1/1 -> Bus Selector/1
  Bus Selector/1 -> Mux/1  "<Righ arm - Overall Translational Movement>"
  Bus Selector/2 -> Mux/2  "<Left arm - Overall Translational Movement>"
  Bus Selector/3 -> Mux/3  "<Camera shell open>"
  Bus Selector/4 -> Mux/4  "<Camera Pan>"
  Bus Selector/5 -> Mux/5  "<Camera Tilt>"

== system irep_force_control_simu/In-Vivo System/D/A/Level 1 ==
  note: Measurement Computing
      | PCI-DDA08/12 Analog Output
      | slot: [2, 7]
  In1 : Inport
  Demux1 : Demux  Outputs=8
  Terminator{,1..7} (8 alike) : Terminator
  wires:
  Demux1/1 -> Terminator/1
  Demux1/2 -> Terminator1/1
  Demux1/3 -> Terminator2/1
  Demux1/4 -> Terminator3/1
  Demux1/5 -> Terminator4/1
  Demux1/6 -> Terminator5/1
  Demux1/7 -> Terminator6/1
  Demux1/8 -> Terminator7/1
  In1/1 -> Demux1/1

== system irep_force_control_simu/In-Vivo System/D/A/Level 2 ==
  note: Measurement Computing
      | PCI-DDA08/12 Analog Output
      | Slot: [2, 10]
  In1 : Inport
  Demux2 : Demux  Outputs=8
  Terminator{,1..7} (8 alike) : Terminator
  wires:
  Demux2/1 -> Terminator/1
  Demux2/2 -> Terminator1/1
  Demux2/3 -> Terminator2/1
  Demux2/4 -> Terminator3/1
  Demux2/5 -> Terminator4/1
  Demux2/6 -> Terminator5/1
  Demux2/7 -> Terminator6/1
  Demux2/8 -> Terminator7/1
  In1/1 -> Demux2/1

== system irep_force_control_simu/In-Vivo System/D/A/Level 3 ==
  note: Measurement Computing
      | PCI-DDA08/12
      | Analog Ouput
      | Slot: [2, 13]
      | Channels [1,4,5,6,7]
  In1 : Inport
  Demux1 : Demux  Outputs=5
  Terminator{,3..6} (5 alike) : Terminator
  wires:
  In1/1 -> Demux1/1
  Demux1/1 -> Terminator/1
  Demux1/2 -> Terminator3/1
  Demux1/3 -> Terminator4/1
  Demux1/4 -> Terminator5/1
  Demux1/5 -> Terminator6/1

== system irep_force_control_simu/In-Vivo System/D/A/Parker Level ==
  note: Measurement Computing
      | PCI-DAS1602/12
      | Analog Output
      | Slot: [1, 14]
  In1 : Inport
  Bus Selector : BusSelector  OutputSignals=Parker insertion stage,Parker rotary stage
  Gain : Gain  Gain=-1
  Gain1 : Gain  Gain=-1
  Terminator : Terminator
  Terminator1 : Terminator
  wires:
  Bus Selector/2 -> Gain/1  "<Parker rotary stage>"
  Bus Selector/1 -> Gain1/1  "<Parker insertion stage>"
  Gain/1 -> Terminator1/1
  Gain1/1 -> Terminator/1
  In1/1 -> Bus Selector/1

== system irep_force_control_simu/In-Vivo System/Loadcells/Loadcell Backbone Mapping ==
  note: This direction gain is needed for the following reason:
      | The load cell reading "+" meaning tension, i.e. pushing on the backbone.
      | Pushing in the statics formulation use "-".
      | So the loadcell sign is opposite to the statics formulation
  note: This mapping is documented on the wiki
      | http://arma.vuse.vanderbilt.edu/mediawiki/index.php/Force_Sensing,_In-Vivo_Project#Loadcell__Backbone_Mapping
  loadcell reading : Inport
  Demux : Demux  Outputs=8
  Mux : Mux  Inputs=8
  direction : Gain  Gain=-1
  tau backbones : Outport
  wires:
  loadcell reading/1 -> Demux/1
  Demux/1 -> [LC1]  "LC1"
  Demux/2 -> [LC2]  "LC2"
  Demux/3 -> [LC3]  "LC3"
  Demux/4 -> [LC4]  "LC4"
  Demux/5 -> [LC5]  "LC5"
  Demux/6 -> [LC6]  "LC6"
  Demux/7 -> [LC7]  "LC7"
  Demux/8 -> [LC8]  "LC8"
  [LC1] -> Mux/1  "Seg1 BB1"
  [LC4] -> Mux/2  "Seg1 BB2"
  [LC2] -> Mux/3  "Seg1 BB3"
  [LC3] -> Mux/4  "Seg1 BB4"
  [LC8] -> Mux/5  "Seg2 BB1"
  [LC5] -> Mux/6  "Seg2 BB2"
  [LC7] -> Mux/7  "Seg2 BB3"
  [LC6] -> Mux/8  "Seg2 BB4"
  Mux/1 -> direction/1
  direction/1 -> tau backbones/1

== system irep_force_control_simu/In-Vivo System/Magnetic Tracker 125 Hz/process trak1 ==
  raw : Inport
  Filter1 : Subsystem
  Gain : Gain  Gain=[25.4 25.4 25.4 1 1 1]  SampleTime=dt_trakstar
  tracker inversion : Gain  Gain=[-1 -1 -1 -1 -1 -1]  SampleTime=dt_trakstar
  trakstar_to_pose : MATLAB Function  TreatAsAtomicUnit=on
  sensor_pose : Outport
  wires:
  Gain/1 -> Filter1/1(in)
  Filter1/1(out) -> trakstar_to_pose/1(u)
  raw/1 -> Gain/1
  trakstar_to_pose/1(sensor) -> tracker inversion/1
  tracker inversion/1 -> sensor_pose/1

== system irep_force_control_simu/In-Vivo System/Magnetic Tracker 125 Hz/process trak2 ==
  raw : Inport
  Filter1 : Subsystem
  Gain : Gain  Gain=[25.4 25.4 25.4 1 1 1]  SampleTime=dt_trakstar
  trakstar_to_pose : MATLAB Function  TreatAsAtomicUnit=on
  sensor_pose : Outport
  wires:
  trakstar_to_pose/1(sensor) -> sensor_pose/1
  raw/1 -> Gain/1
  Filter1/1(out) -> trakstar_to_pose/1(u)
  Gain/1 -> Filter1/1(in)

== system irep_force_control_simu/In-Vivo System/Magnetic Tracker 125 Hz/process trak3 ==
  raw : Inport
  Filter1 : Subsystem
  Gain : Gain  Gain=[25.4 25.4 25.4 1 1 1]  SampleTime=dt_trakstar
  trakstar_to_pose : MATLAB Function  TreatAsAtomicUnit=on
  sensor_pose : Outport
  wires:
  Gain/1 -> Filter1/1(in)
  Filter1/1(out) -> trakstar_to_pose/1(u)
  raw/1 -> Gain/1
  trakstar_to_pose/1(sensor) -> sensor_pose/1

== system irep_force_control_simu/In-Vivo System/Magnetic Tracker 125 Hz/process trak4 ==
  raw : Inport
  Filter1 : Subsystem
  Gain : Gain  Gain=[25.4 25.4 25.4 1 1 1]  SampleTime=dt_trakstar
  trakstar_to_pose : MATLAB Function  TreatAsAtomicUnit=on
  sensor_pose : Outport
  wires:
  trakstar_to_pose/1(sensor) -> sensor_pose/1
  raw/1 -> Gain/1
  Filter1/1(out) -> trakstar_to_pose/1(u)
  Gain/1 -> Filter1/1(in)

== system irep_force_control_simu/In-Vivo System/Potentiometers/Filter ==
  in : Inport
  Discrete FIR Filter : DiscreteFir  CoefSource=Input port  AccumDataTypeStr=Inherit: Same as product output
  Gain : Gain  Gain=1/N_pots
  vel_filter_coeffs : Constant  Value=pots_filter_coeffs
  out : Outport
  wires:
  in/1 -> Discrete FIR Filter/1
  Gain/1 -> out/1
  vel_filter_coeffs/1 -> Discrete FIR Filter/2
  Discrete FIR Filter/1 -> Gain/1

== system irep_force_control_simu/In-Vivo System/Potentiometers/Filter1 ==
  in : Inport
  Discrete FIR Filter : DiscreteFir  CoefSource=Input port  AccumDataTypeStr=Inherit: Same as product output
  Gain : Gain  Gain=1/N_pots
  vel_filter_coeffs : Constant  Value=pots_filter_coeffs
  out : Outport
  wires:
  Discrete FIR Filter/1 -> Gain/1
  vel_filter_coeffs/1 -> Discrete FIR Filter/2
  Gain/1 -> out/1
  in/1 -> Discrete FIR Filter/1

== system irep_force_control_simu/In-Vivo System/Potentiometers/Filter2 ==
  in : Inport
  Discrete FIR Filter : DiscreteFir  CoefSource=Input port  AccumDataTypeStr=Inherit: Same as product output
  Gain : Gain  Gain=1/N_pots
  vel_filter_coeffs : Constant  Value=pots_filter_coeffs
  out : Outport
  wires:
  Discrete FIR Filter/1 -> Gain/1
  vel_filter_coeffs/1 -> Discrete FIR Filter/2
  Gain/1 -> out/1
  in/1 -> Discrete FIR Filter/1

== system irep_force_control_simu/In-Vivo System/Potentiometers/Filter3 ==
  in : Inport
  Discrete FIR Filter : DiscreteFir  CoefSource=Input port  AccumDataTypeStr=Inherit: Same as product output
  Gain : Gain  Gain=1/N_joystick
  vel_filter_coeffs : Constant  Value=joystick_filter_coeffs
  out : Outport
  wires:
  in/1 -> Discrete FIR Filter/1
  Gain/1 -> out/1
  vel_filter_coeffs/1 -> Discrete FIR Filter/2
  Discrete FIR Filter/1 -> Gain/1

== system irep_force_control_simu/In-Vivo System/Potentiometers/Initialize Joystick ==
  In1 : Inport
  Digital Clock : DigitalClock  SampleTime=dt
  Embedded MATLAB Function : MATLAB Function  TreatAsAtomicUnit=on
  Unit Delay : UnitDelay  InitialCondition=zeros(3,1)  SampleTime=dt
  Out1 : Outport
  wires:
  Digital Clock/1 -> Embedded MATLAB Function/2(t)
  Unit Delay/1 -> Embedded MATLAB Function/3(u_prev)
  In1/1 -> Embedded MATLAB Function/1(u_curr)
  Embedded MATLAB Function/1(V) -> Out1/1  "camer"
  Embedded MATLAB Function/2(v_zero) -> Unit Delay/1  "camera joystick"

== system irep_force_control_simu/In-Vivo System/motor simulation/Bus Creator ==
  In1 : Inport
  Bus Creator : BusCreator  Inputs=23
  Demux : Demux  Outputs=23
  Out1 : Outport
  wires:
  Demux/23 -> Bus Creator/23  "Parker rotary stage"
  Demux/22 -> Bus Creator/22  "Parker insertion stage"
  In1/1 -> Demux/1
  Bus Creator/1 -> Out1/1
  Demux/21 -> Bus Creator/21  "Camera Tilt"
  Demux/20 -> Bus Creator/20  "Camera Pan"
  Demux/19 -> Bus Creator/19  "Camera shell open"
  Demux/18 -> Bus Creator/18  "Left arm - overall translational movement"
  Demux/17 -> Bus Creator/17  "Right arm - overall translational movement"
  Demux/16 -> Bus Creator/16  "Left arm - parallelogram insert joint"
  Demux/15 -> Bus Creator/15  "Left arm - parallelogram deployment joint"
  Demux/14 -> Bus Creator/14  "Left arm - distal segment - bending in y"
  Demux/13 -> Bus Creator/13  "Left arm - wrist"
  Demux/12 -> Bus Creator/12  "Left arm - distal segment - bending in x"
  Demux/11 -> Bus Creator/11  "Left arm - proximal segment - bending in X"
  Demux/10 -> Bus Creator/10  "Left arm - gripper joint"
  Demux/9 -> Bus Creator/9  "Left arm - proximal segment - bending in Y"
  Demux/8 -> Bus Creator/8  "Right arm - parallelogram insert joint"
  Demux/7 -> Bus Creator/7  "Right arm - parallelogram deployment joint"
  Demux/6 -> Bus Creator/6  "Right arm - distal segment - bending in Y"
  Demux/5 -> Bus Creator/5  "Right arm - wrist"
  Demux/4 -> Bus Creator/4  "Right arm - distal segment - bending in X"
  Demux/3 -> Bus Creator/3  "Right arm - Proximal segment - bending in X"
  Demux/2 -> Bus Creator/2  "Right arm - Gripper Joint"
  Demux/1 -> Bus Creator/1  "Righ arm - Proximal segment - bending in Y"

== system irep_force_control_simu/In-Vivo System/motor simulation/motor simu ==
  u : Inport
  Discrete-Time Integrator : DiscreteIntegrator  InitialCondition=zeros(23,1)  SampleTime=dt
  Discrete-Time Integrator1 : DiscreteIntegrator  InitialCondition=zeros(23,1)  SampleTime=dt
  Gain : Gain  Gain=1./B_simu
  q cur : Outport
  wires:
  Gain/1 -> Discrete-Time Integrator/1
  u/1 -> Gain/1
  Discrete-Time Integrator1/1 -> q cur/1
  Discrete-Time Integrator/1 -> Discrete-Time Integrator1/1

== system irep_force_control_simu/In-Vivo System/motor simulation/q_des to q_cur mapping ==
  q cur in : Inport
  Bus Creator1 : BusCreator  Inputs=23
  Bus Selector : BusSelector  OutputSignals=Right arm - Proximal Segment Y,Right arm - Gripper Joint,Right arm - Proximal Segment X,Right arm - Distal Segment X,Right arm - Wrist Joint,Right arm - Distal Segment Y,Right arm - Parallelogram Deploy,Right arm - Parallelogram Insert,Left arm - Proximal Segment Y,Left arm - Gripper Joint,Left arm - Proximal Segment X,Left arm - Distal Segment X,Left arm - Wrist Joint,Left arm - Distal Segment Y,Left arm - Parallelogram Deploy,Left arm - Parallelogram Insert,Righ arm - Overall Translational Movement,Left arm - Overall Translational Movement,Camera shell open,Camera Pan,Camera Tilt,Parker insertion stage,Parker rotary stage
  Demux : Demux  Outputs=23
  Mux : Mux  Inputs=23
  q cur out : Outport
  wires:
  Demux/1 -> Bus Creator1/1  "Righ arm - Overall Translational Movement"
  Demux/2 -> Bus Creator1/2  "Right arm - Parallelogram Insert"
  Demux/3 -> Bus Creator1/3  "Right arm - Parallelogram Deploy"
  Demux/4 -> Bus Creator1/4  "Right arm - Proximal Segment X"
  Demux/5 -> Bus Creator1/5  "Right arm - Proximal Segment Y"
  Demux/6 -> Bus Creator1/6  "Right arm - Distal Segment X"
  Demux/7 -> Bus Creator1/7  "Right arm - Distal Segment Y"
  Demux/8 -> Bus Creator1/8  "Right arm - Wrist Joint"
  Demux/9 -> Bus Creator1/9  "Right arm - Gripper Joint"
  Demux/10 -> Bus Creator1/10  "Left arm - Overall Translational Movement"
  Demux/11 -> Bus Creator1/11  "Left arm - Parallelogram Insert"
  Demux/12 -> Bus Creator1/12  "Left arm - Parallelogram Deploy"
  Demux/13 -> Bus Creator1/13  "Left arm - Proximal Segment X"
  Demux/14 -> Bus Creator1/14  "Left arm - Proximal Segment Y"
  Demux/15 -> Bus Creator1/15  "Left arm - Distal Segment X"
  Demux/16 -> Bus Creator1/16  "Left arm - Distal Segment Y"
  Demux/17 -> Bus Creator1/17  "Left arm - Wrist Joint"
  Demux/18 -> Bus Creator1/18  "Left arm - Gripper Joint"
  Demux/19 -> Bus Creator1/19  "Camera shell open"
  Demux/20 -> Bus Creator1/20  "Camera Pan"
  Demux/21 -> Bus Creator1/21  "Camera Tilt"
  Demux/22 -> Bus Creator1/22  "Parker insertion stage"
  Demux/23 -> Bus Creator1/23  "Parker rotary stage"
  Bus Creator1/1 -> Bus Selector/1
  Bus Selector/1 -> Mux/1  "<Right arm - Proximal Segment Y>"
  Bus Selector/2 -> Mux/2  "<Right arm - Gripper Joint>"
  Bus Selector/3 -> Mux/3  "<Right arm - Proximal Segment X>"
  Bus Selector/4 -> Mux/4  "<Right arm - Distal Segment X>"
  Bus Selector/5 -> Mux/5  "<Right arm - Wrist Joint>"
  Bus Selector/6 -> Mux/6  "<Right arm - Distal Segment Y>"
  Bus Selector/7 -> Mux/7  "<Right arm - Parallelogram Deploy>"
  Bus Selector/8 -> Mux/8  "<Right arm - Parallelogram Insert>"
  Bus Selector/9 -> Mux/9  "<Left arm - Proximal Segment Y>"
  Bus Selector/10 -> Mux/10  "<Left arm - Gripper Joint>"
  Bus Selector/11 -> Mux/11  "<Left arm - Proximal Segment X>"
  Bus Selector/12 -> Mux/12  "<Left arm - Distal Segment X>"
  Bus Selector/13 -> Mux/13  "<Left arm - Wrist Joint>"
  Bus Selector/14 -> Mux/14  "<Left arm - Distal Segment Y>"
  Bus Selector/15 -> Mux/15  "<Left arm - Parallelogram Deploy>"
  Bus Selector/16 -> Mux/16  "<Left arm - Parallelogram Insert>"
  Bus Selector/17 -> Mux/17  "<Righ arm - Overall Translational Movement>"
  Bus Selector/18 -> Mux/18  "<Left arm - Overall Translational Movement>"
  Bus Selector/19 -> Mux/19  "<Camera shell open>"
  Bus Selector/20 -> Mux/20  "<Camera Pan>"
  Bus Selector/21 -> Mux/21  "<Camera Tilt>"
  Bus Selector/22 -> Mux/22  "<Parker insertion stage>"
  Bus Selector/23 -> Mux/23  "<Parker rotary stage>"
  q cur in/1 -> Demux/1
  Mux/1 -> q cur out/1
